simulink model "bh_test_car_viewer"  (R2017b)
settings: Solver=ode45  StartTime=0.0  StopTime=10  FixedStep=0.001  RelTol=1e-5
libraries: bh_cv_car_drc_library x1
settings Model: Creator=bhorton  LastModifiedBy=bhorton
settings SolverCC: ZeroCrossControl=EnableAll  ZeroCrossAlgorithm=Adaptive
settings DebuggingCC: SignalInfNanChecking=warning
settings ModelReferenceCC: ModelReferenceMinAlgLoopOccurrences=on

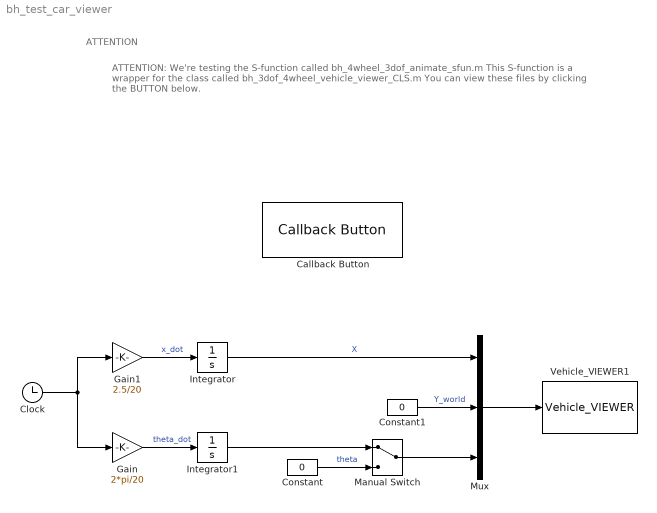
== system bh_test_car_viewer ==
  note: ATTENTION
  note: ATTENTION:
      |
      | We're testing the S-function called bh_4wheel_3dof_animate_sfun.m
      |
      | This S-function is a wrapper for the class called bh_3dof_4wheel_vehicle_viewer_CLS.m
      |
      | You can view these files by clicking the BUTTON below.
  Callback Button : CallbackButton  WebBlockId=1627  ButtonText=View M-files  PressDelay=500  RepeatInterval=0
      settings: ClickFcn=|
      | edit('bh_4wheel_3dof_animate_sfun.m', ...
      |      'bh_3dof_4wheel_vehicle_viewer_CLS.m')
  Clock : Clock
  Constant : Constant  Value=0
  Constant1 : Constant  Value=0
  Gain : Gain  Gain=2*pi/20
  Gain1 : Gain  Gain=2.5/20
  Integrator : Integrator
  Integrator1 : Integrator
  Manual Switch : ManualSwitch
  Mux : Mux  Inputs=3
  Vehicle_VIEWER1 : bh_cv_car_drc_library/CAR_things/Vehicle_VIEWER  wp_mat=[-1, -1; 2,2]  veh_ID_num=1  veh_init_xytheta=[0,0,0]  Ts=0.1
  wires:
  Constant1/1 -> Mux/2  "Y_world"
  Constant/1 -> Manual Switch/2  "theta"
  Integrator/1 -> Mux/1  "X"
  Clock/1 -> Gain/1, Gain1/1
  Manual Switch/1 -> Mux/3
  Mux/1 -> Vehicle_VIEWER1/1
  Gain1/1 -> Integrator/1  "x_dot"
  Gain/1 -> Integrator1/1  "theta_dot"
  Integrator1/1 -> Manual Switch/1
